simulink model "AV10_Z1"  (R2018a)
settings: Solver=VariableStepAuto  StartTime=0.0  StopTime=2000  RelTol=1e-3
values from neighbouring files (symbols this model uses):
  q0 = -1.1901    [AV10_ZADACHA1.m]    (also in AV9_PRIMER2_VREDNOSTI.m = -62.3782; AV9_PRIMER4.m = 1.9573; AV9_PRIMER5.m = 1.8649; AV_10_PRIMER1.m = 1.512)
  q1 = 0.8945    [AV10_ZADACHA1.m]    (also in AV9_PRIMER2_VREDNOSTI.m = 122.0694; AV9_PRIMER4.m = -1.6594; AV9_PRIMER5.m = -1.8649; AV_10_PRIMER1.m = -1.423)
  q2 = -0.2805    [AV10_ZADACHA1.m]    (also in AV9_PRIMER2_VREDNOSTI.m = -59.9743; AV9_PRIMER4.m = 0.6675; AV9_PRIMER5.m = 0.2403; AV_10_PRIMER1.m = 0.44)
  T = 160    [AV10_ZADACHA1.m]    (also in AV9_PRIMER4.m = 16; AV9_PRIMER5.m = 4; AV_10_PRIMER1.m = 8)
settings Model: Creator=DD  LastModifiedBy=DD

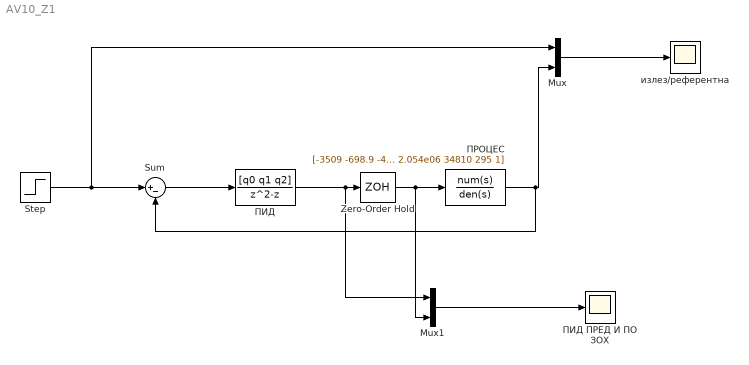
== system AV10_Z1 ==
  Mux : Mux  Inputs=2
  Mux1 : Mux  Inputs=2
  Step : Step  SampleTime=0
  Sum : Sum  Inputs=|+-
  Zero-Order Hold : ZeroOrderHold  SampleTime=-1
  ПИД : DiscreteTransferFcn  Numerator=[q0 q1 q2]  Denominator=[1 -1 0]  SampleTime=T
  "ПИД ПРЕД И ПО ЗОХ " : Scope
  ПРОЦЕС : TransferFcn  Numerator=[-3509 -698.9 -46.02 -1]  Denominator=[7.149e08 6.059e07 2.054e06 34810 295 1]
  излез/референтна : Scope
  wires:
  Step/1 -> Mux/1, Sum/1
  Sum/1 -> ПИД/1
  ПИД/1 -> Mux1/1, Zero-Order Hold/1
  Zero-Order Hold/1 -> Mux1/2, ПРОЦЕС/1
  ПРОЦЕС/1 -> Sum/2, Mux/2
  Mux/1 -> излез/референтна/1
  Mux1/1 -> "ПИД ПРЕД И ПО ЗОХ "/1
